simulink model "combinedTxRx_16bit"  (R2017a)
settings: Solver=FixedStepDiscrete  StartTime=0.0  StopTime=10.0  RelTol=1e-3
InitFcn:
  | numHeaderBits = 16;
  | %numPreambleBits = 250;
  | AGCBarkerSymbols = 160+28;
  | EQTrainingSymbols = 250;
  | CRCGeneratorLag = 34; % CRCLen + 2
  | 
  | %% AGC Preamble
  | B13bipolar = [0 0 0 0 0 2 2 0 0 2 0 2];
  | rep = [B13bipolar, B13bipolar(1:4)];
  | AGCBarker = repmat(rep,1,10);
  | % Second preamble part
  | B11bipolar = [0 0 0 2 2 2 0 2  2 0 2];
  | TimingBarker = [B11bipolar,B11bipolar,B11bipolar,B11bipolar(1:6)];
  | PreambleBarkersInts = [AGCBarker, TimingBarker];
  | % Convert integer into their bit representation
  | PreambleBarkersBits = zeros(1,length(PreambleBarkersInts)*2);
  | PreambleBarkersBits(1:2:end) = (PreambleBarkersInts==2);
  | 
  | % Constants
  | % First preamble part
  | B13bipolar = [0 0 0 0 0 2 2 0 0 2 0 2];
  | rep = [B13bipolar, B13bipolar(1:4)];
  | AGCBarker = repmat(rep,1,10);
  | % Second preamble part
  | B11bipolar = [0 0 0 2 2 2 0 2  2 0 2];
  | TimingBarker = [B11bipolar,B11bipolar,B11bipolar(1:6)];
  | PreambleBarkersInts = [AGCBarker, TimingBarker];
  | % Convert integer into their bit representation
  | PreambleBarkersBits = false(1,length(PreambleBarkersInts)*2);
  | PreambleBarkersBits(1:2:end) = logical(PreambleBarkersInts==2);
  | pLen = uint16(length(PreambleBarkersBits));
  | 
  | 
  | %%%%%%%%%%%%%%%%%%%%%%%%%%
  | %% RX
  | %%%%%%%%%%%%%%%%%%%%%%%%%%
  | 
  | barker = comm.BarkerCode('SamplesPerFrame', 28, 'Length', 11);
  | seq = barker()+1;
  | M = 4;
  | hPSKModTrain   = comm.PSKModulator(M, ...
  |     'PhaseOffset',pi/4, ...
  |     'SymbolMapping','Binary');
  | xPreambleSeq = hPSKModTrain(seq);
  | 
  | 
  | %%%%%%%%%%%%
  | 
  | % AGC Preamble
  | reps = 5;
  | barker = comm.BarkerCode('SamplesPerFrame', 16, 'Length', 13);
  | seq = barker()+1;
  | %preamble = zeros(16*reps,1);
  | preambleFull = repmat(seq,reps,1);
  | rctFilt = comm.RaisedCosineTransmitFilter('FilterSpanInSymbols', 128,...
  | 'RolloffFactor',0.5,...
  | 'OutputSamplesPerSymbol',4);
  | preambleFullFilt = rctFilt(preambleFull);
  | 
  | %%%%%%%%%%%%
  | ... (+26 lines)
undefined symbols (not defined in the file or in its folder): j
libraries: simulink x22, dsphdlfiltering x20, hdlsllib x6, commseqgen3 x4, dspsigops x4, commdigbbndpm3 x3, commcrc2 x2, commcnvcod2 x2, dspstat3 x2, commsource2 x1, commutil2 x1, commfilt2 x1
(part 3 of 3)

== matlab function combinedTxRx_16bit/Combined TX and RX/Tx Under Test/Transmitter HDL/Packet Generation/Tx Controller ==
  data: modeOut output; headerData output; data output; payloadBit input; payloadSize input; count input; start input; dataStart output; dataEnd output; preambleReset output
function [modeOut, headerData, data, dataStart, dataEnd, preambleReset] = fcn(payloadBit,payloadSize,count, start)

% When we get a start flag buffers are reset and the next cycle with start
% in mode 0

% Reset: New payload size is passed at an int16
% 


persistent  headerBits numPayloadBits mode

numHeaderBits = uint32(16);
AGCBarkerSymbols = 160+28;
EQTrainingSymbols = 250; % 2 bits per symbol => 250 symbols
preambleBits = uint32(EQTrainingSymbols+AGCBarkerSymbols-0);
CRCLength = 32;
CRCGeneratorLag = CRCLength+2+0; % additional 1 is from reset of encoder
CodeRate = 2;
lagBits = 40+68;

% Async/Init
if isempty(numPayloadBits)
    % Sizes of frame sections
    numPayloadBits = uint32(0); 
    %headerBits = zeros(1,numHeaderBits)>0;
    headerBits = uint16(0);
    mode = uint8(4);
end

% Synchronous
switch mode
    case uint8(0) % Reset
        % Move to next mode on next input/clock
        mode = uint8(1);
        % Convert payloadSize to bits
        numPayloadBits = uint32(bitshift(payloadSize,3)+CRCLength);
        %headerBits = logical(bitget(CodeRate*(payloadSize+CRCLength),1:numHeaderBits));
        headerBits = uint16(bitshift((bitshift(payloadSize,3)+CRCLength+lagBits),1));        
        % Set outputs
        modeOut = uint8(4);
        headerData = false;
        data = false; % Not used downstream
        dataStart = false;
        dataEnd = false;
        preambleReset = true;
    case uint8(1) % Preamble
        % Set Next Mode
        if count>=(preambleBits)
            preambleReset = false;
            mode = uint8(2);
        elseif count==uint32(1)
            preambleReset = false;
            mode = uint8(1);
        else
            preambleReset = false;
            mode = uint8(1);
        end
        % Set outputs
        modeOut = uint8(1);
        headerData = false;
        % Start outputing data early to compensate for CRC lag
        if count>=(preambleBits+numHeaderBits-CRCGeneratorLag)
           data = payloadBit;
           % Set flag on first payload bit
           dataStart = count == (preambleBits+numHeaderBits-CRCGeneratorLag);
        else
           data = false;         
           dataStart = false;
        end
        dataEnd = false;
    case uint8(2) % Header bits
        % Set Next Mode
        if count>=(preambleBits+numHeaderBits)
            mode = uint8(3);
        else
            mode = uint8(2);
        end
        % Set outputs
        modeOut = uint8(2);
        %headerData = headerBits(count-preambleBits);
        headerData = bitget(headerBits,count-preambleBits)>0;
        data = payloadBit;
        dataStart = false;
        dataEnd = false;
        preambleReset = false;
    case uint8(3) % Payload bits and CRC
        % Set Next Mode
        if count>=(preambleBits+numHeaderBits+numPayloadBits)%+CRCGeneratorLag)
            % Will coencide with last CRC Bit
            mode = uint8(4);
        else
            mode = uint8(3);
        end
        % Set outputs
        modeOut = uint8(3);        
        headerData = false;
        data = payloadBit;
        % Set flag on last payload bit
        dataStart = false;
        dataEnd =   ( count==(preambleBits+numHeaderBits+numPayloadBits-CRCLength-CRCGeneratorLag-1) );
        preambleReset = false;
    otherwise %case uint8(4) % Waiting for data
        % Chilling for new start
        if start
           mode = uint8(0); 
        else
           mode = uint8(4);
        end
        % Set outputs
        modeOut = uint8(4);
        headerData = false;
        data = false; % Not used downstream
        dataStart = false;
        dataEnd = false;
        preambleReset = false;
end

== matlab function combinedTxRx_16bit/Combined TX and RX/Tx Under Test/Transmitter HDL/DMA Interface/DMA Control ==
  data: byteIn input; bitOut output; validIn input; validOut output; startOut output; payloadLength output; readyForInput output; EOF input
function [bitOut,validOut,startOut,payloadLength,readyForInput] = DMA_Control(byteIn,validIn,EOF)

% This block converts the byte input pipeline into bits and extract the
% length the packet into its own signal

persistent wordBuffer bitCounter payloadLenBuff mode inputByteCounter

bitsInInput = uint8(16);

if isempty(wordBuffer)
    wordBuffer = uint16(0); % Must match number of bits defined by bitsInInput
    bitCounter = uint8(0);
    payloadLenBuff = uint16(0);
    mode = uint8(0);
    inputByteCounter = uint16(0);
end

%% Payload length setup
% Capture first payload length byte(s)
if validIn && mode == uint8(0)
    bitOut = false;
    validOut = false;
    startOut = true;
    payloadLength = uint16(0);
    readyForInput = true;
    mode = uint8(2);
    inputByteCounter = uint16(0);% Reset
    
    %payloadLenBuff = bitshift(uint16(byteIn),8); % Place upper bits first
    payloadLenBuff = uint16(byteIn); 
    

%% Payload output
% Byte edge of data
elseif validIn && (mode==uint8(2))
    bitOut = bitget(byteIn,1)>0;
    wordBuffer = byteIn; % Save byte
    bitCounter = uint8(2);% Reset
    validOut = true;
    startOut = false;
    readyForInput = false;
    payloadLength = uint16(payloadLenBuff);
    % Bytes processed
    inputByteCounter = inputByteCounter + uint16(bitsInInput/8);    
    
% Remaining N-1 bits of input byte(s)
elseif (bitCounter > uint8(0))  && (mode==uint8(2))
    bitOut = bitget(wordBuffer,bitCounter)>0;
    startOut = false;
    payloadLength = uint16(payloadLenBuff);
    validOut = true;
    if bitCounter >= uint8(bitsInInput)
        bitCounter = uint8(0);
        % If we've processed all the bytes we need to wait for downstream
        % to be done
        if inputByteCounter<payloadLenBuff
            readyForInput = true; % Tell them we need next byte
        else
            readyForInput = false; % Hold DMA off for now, next call will go to EOF
            mode = uint8(3);
        end
    else
        bitCounter = bitCounter+uint8(1);
        readyForInput = false;
    end
% Waiting for EOF from packet generation
elseif (mode==uint8(3))
    bitOut = false;
    validOut = true; % Keep downstream processing going
    startOut = false;
    payloadLength = uint16(payloadLenBuff);
    if EOF % Done with frame now ask for more data
        readyForInput = true;
        mode = uint8(0);% Reset
    else
        readyForInput = false;
    end
    
else % not-valid and need another byte
    bitOut = false;
    if mode == uint8(0)
        validOut = true; % Let LFSR Run
    else
        validOut = false;
    end
    startOut = false;
    payloadLength = uint16(0);
    readyForInput = true;
end

== matlab function combinedTxRx_16bit/Combined TX and RX/Tx Under Test/Transmitter HDL/Packet Generation/Payload/HDL Scrambler 2 bits/Buffer Manage ==
  data: bit1 input; bit2 input; outBuffer output; reset input
function outBuffer = fcn(bit1, bit2, reset)
%#codegen

init_buffer = logical([0 1 0 0 0 1 0]);

persistent buffer

if isempty(buffer)
    buffer = init_buffer;
end

if reset
    outBuffer = init_buffer;
    buffer = init_buffer;
    %outBuffer = [init_buffer(3:end),bit1,bit2];
    %buffer = [buffer(3:end),bit1,bit2];    
else
    outBuffer = [bit2,bit1,buffer(1:end-2)];
    buffer = [bit2,bit1,buffer(1:end-2)];
end

== matlab function combinedTxRx_16bit/Combined TX and RX/Tx Under Test/DMA Model Driver ==
  data: driver input; payload output; valid output boolean; enable input
function [payload,valid] = fcn(driver, enable)
%#codegen

persistent indx mode

pSize = uint16(200); % Size in bytes (Must be multiple of 32 bits) cannot exceed uint16 max
mask = uint16(sum(2.^(0:15)));

if isempty(indx)
    indx = pSize;
    mode = int8(0);
end

% % Randomly dont transmit new data
% if enable && mode == 0
%    enable = randn>1; 
% end

if enable && driver
    valid = true;
    switch mode
        case int8(0) % Fresh packet start
%             disp('New Packet Start');
            payload = uint16(pSize);%Upper bits
            mode = int8(1);
            indx = uint16(0);
        otherwise%case 2
            indx = indx + uint16(2);
            %payload = uint32(sum(2.^[0 2 4 6 8 10 12 14 ]));
            payload = uint16(21845);%sum(2.^[0:2:14])); % Alternating ones and zeros
            if indx == pSize % reached end of frame
                mode = int8(0);
            end
    end
else
    valid = false;
    payload = uint16(0);
end

== matlab function combinedTxRx_16bit/Combined TX and RX/Receiver HDL/CRC Check and DMA Pack/CRC Check ES/Check CRC Result (DEBUG) ==
  data: bits input; start input; done input; valid input; err input
function fcn(bits, start, done, valid, err)

persistent buffer

if isempty(buffer)
    buffer = fi(false(1032,1),0,1,0);
end

buffer = [buffer(2:end);bits];

if done && valid
    if err
        fprintf('CRC Error (HDL CRC)\n');
    else
        fprintf('CRC Passed (HDL CRC)\n');
    end
end
if err % Flag if any error every occurs, if it occurs alone it means given crc is not long enough
    fprintf('CRC Error Type 2 (HDL CRC)\n');
end

== matlab function combinedTxRx_16bit/Combined TX and RX/Receiver HDL/CRC Check and DMA Pack/CRC Check ES/Debug CRC input ==
  data: u input; enable input; endFlag input; startFlag input
function fcn(u, enable,endFlag,startFlag)

persistent buffer crc count

if isempty(buffer)
   buffer = false(1700,1); 
    crc = comm.CRCDetector('Polynomial','z^32 + z^26 + z^23 + z^22 + z^16 + z^12 + z^11 + z^10 + z^8 + z^7 + z^5 + z^4 + z^2 + z + 1');
    count = 1;
end

if enable
    %buffer = [buffer(2:end);u];
    if startFlag
        count = 1;
    elseif count>1700-1
        count = 1;
    else
        count = count + 1;
    end
    buffer(count) = u;
    
    if endFlag
        disp(count)
        k = buffer(1:1632);
        [~,e] = crc(k);
        if e
            disp('Error');
        else
            disp('Pass');
        end
    end
    
end

== matlab function combinedTxRx_16bit/Combined TX and RX/Receiver HDL/CRC Check and DMA Pack/DMA Interface/Bit Packer ==
  data: bitIn input; byteOut output; startIn input; endIn input; err input; validIn input; validOut output; startOut output
function [byteOut,validOut,startOut] = BitPacker(bitIn, startIn, endIn, err, validIn)

% This block will pack bits into bytes with start boundaries


% Constants
bits2Pack = uint8(16); % byteReg must contain this many bits
% NOTE: Frames but be a multiple of bits2Pack or bits will be trimmed from
% end

persistent byteReg byteIndx setStartFlag

if isempty(byteIndx)
    byteReg  = uint16(0);
    byteIndx = uint8(1);
    setStartFlag = false;
end

if validIn
    if startIn % Reset
        bitset(byteReg,1,bitIn);
        byteIndx = uint8(2);
        validOut = false;
        setStartFlag = true;
        startOut = false;
    else
        byteReg = bitset(byteReg,byteIndx,bitIn);
        if byteIndx >= bits2Pack
            byteIndx = uint8(1);
            validOut = true;
            startOut = setStartFlag;
            setStartFlag = false;
        else
            byteIndx = byteIndx + uint8(1);
            validOut = false;
            startOut = false;
        end
    end
elseif endIn % Append error bit to last byte
    byteReg = uint16(err);
    validOut = true;
    startOut = false;
else
    validOut = false;
    startOut = false;
end

byteOut = byteReg;

== matlab function combinedTxRx_16bit/Combined TX and RX/Receiver HDL/CRC Check and DMA Pack/overdrive ==
  data: validIn input; enableCRC output; endIn input
function enableCRC = fcn(validIn,endIn)

% This block drives the enabled subsystem and additional step so the
% outputs do not stay high but reset.  All signals are reset since the
% driving valid signal is false

persistent gotEndOut

if isempty(gotEndOut)
    gotEndOut = false;
end
    
if validIn
    enableCRC = true;
    gotEndOut = false;
else
    if endIn
        gotEndOut = true;
        enableCRC = true;
    elseif gotEndOut
        enableCRC = true;
    else
        enableCRC = false;
    end
end

== matlab function combinedTxRx_16bit/Combined TX and RX/Receiver HDL/Descramble and Decode/Find packet tail and check CRC (DEBUG ONLY) ==
  data: u input; enable output; crcCase output
function [enable, crcCase]=findTail(u)

persistent tailBits buffer counter head

if isempty(tailBits)
   tailBits = repmat(uint8([1 0 1 1 0 0 1 1 1 1].'),4,1);
   buffer = uint8(zeros(size(tailBits)));
    counter = 0;
    head = uint8(ones(16,1));
end

%buffer = [u; buffer(1:end-1)];
buffer = [buffer(2:end); u];
counter = counter + 2; % Coded bit counter

% Check for tail sequence
found = 0;
if isequal(buffer,tailBits)
   fprintf('Found tail after %d coded bits\n',int64(counter));
   counter = 0;
   found = 1;
end

%% CHECK CRC
persistent crc buffer2
CRCLen = 32;
nPayLoad = 8*200;
nTB = length(tailBits);

if isempty(crc)
    crc = comm.CRCDetector('Polynomial','z^32 + z^26 + z^23 + z^22 + z^16 + z^12 + z^11 + z^10 + z^8 + z^7 + z^5 + z^4 + z^2 + z + 1');
    buffer2 = false(CRCLen+nPayLoad+nTB,1);%false(10532+40,1);
end

crcCase = 0;
enable = false;

buffer2 = [buffer2(2:end); u>0];
%if isequal(head, buffer2(end-15:end))
%   fprintf('Head FOUND %d\n',int64(counter));
%end
if found>0
    NoTailBits = buffer2(1:end-nTB);
    PayloadWithCRC= NoTailBits(end-nPayLoad-CRCLen+1:end);
    enable = true;
    [~,e] = crc(PayloadWithCRC);
    if ~e
        crcCase = 1;
        fprintf('Packet CRC Passed\n');
    else
        crcCase = 0;
        fprintf('Packet CRC Failed\n');
    end
    
end

== matlab function combinedTxRx_16bit/Combined TX and RX/Receiver HDL/Frame Recover/Enable Equalizer and Packet Decode (Latch) ==
  data: start input; enable output; validIn input
function enable = Counter(start,validIn)

persistent count maxCount lastEOF

if isempty(count)
    count = uint32(0);
    maxCount = uint32(2^16); % Largest possible packet length
    lastEOF = false;
end

eof = false;

if validIn
    % Got a barker preamble start allowing data into equalizer
    if start
        count = maxCount;
    end
    
    % Check on change from true to false
    if lastEOF && ~eof
        %     fprintf('Frame end reached\n');
        count = uint32(0);
    end
    lastEOF = eof;
    
    % Past end of max frame size
    if count>0
        count = count - uint32(1);
    end
    
    % Enable downstream
    enable = count>uint32(0);
else
    enable = false;
end

== matlab function combinedTxRx_16bit/Combined TX and RX/Receiver HDL/Frame Recover/Equalization and Demodulation/2 Bit Descrambler/MATLAB Function ==
  data: bits input; bufferA output; reset input; bufferB output
function [bufferA, bufferB] = BufferSelect(bits,reset)

persistent buffer

% Constants
initBuffer = logical([0 1 0 0 0 1 0]);

% Async
if isempty(buffer)
    buffer = initBuffer;
end

% Reset/Sync
if reset
    bufferA = initBuffer;
    bufferB = [bits(1),initBuffer(1:end-1)];
    buffer = [bits(2),bits(1),initBuffer(1:end-2)];
else
    bufferA = buffer;
    bufferB = [bits(1),buffer(1:end-1)];
    buffer = [bits(2),bits(1),buffer(1:end-2)];    
end

== matlab function combinedTxRx_16bit/Combined TX and RX/Receiver HDL/Frame Recover/Equalization and Demodulation/DFE/Equalizer ==
  data: trigger input; eqOut output; data input; trainingSymbol input
function eqOut  = dfe(trigger,data,trainingSymbol)

persistent inputBuffer decisionBuffer forwardTaps backwardTaps processedSamples


%% Constants
WL = uint8(16); FL = uint8(14);
F = fimath('SumMode','SpecifyPrecision','SumWordLength',WL,...
    'SumFractionLength',FL);
% Initial delay guess
channelDelay = uint8(0);
% Equalizer settings
mu = fi(0.05,0,10,12);
nFTaps = uint8(11);
nBTaps = uint8(3);
numTrainingSymbols = uint16(250);
resetTaps = fi([complex(zeros(nFTaps-1,1));1],1,WL,FL,F);

%% Async
if isempty(inputBuffer)
    % Set Precisions
    inputBuffer = fi(complex(zeros(nFTaps,1)),1,WL,FL,F);
    decisionBuffer = fi(complex(zeros(nBTaps,1)),1,WL,FL,F);
    forwardTaps = fi(complex(zeros(nFTaps,1)),1,WL,FL,F);
    backwardTaps = fi(complex(zeros(nBTaps,1)),1,WL,FL,F);
    processedSamples = numTrainingSymbols + uint16(1); % Force to DD mode to start
end

%% Reset
if trigger
    processedSamples = uint16(0);
    % Reset taps
    %forwardTaps = fi(complex(zeros(nFTaps,1)),1,WL,FL,F);
    %forwardTaps(nFTaps-channelDelay) = fi(1,1,WL,FL); % Favor specific delay (causes equalizer to converge faster)
    forwardTaps = resetTaps;
    backwardTaps = fi(complex(zeros(nBTaps,1)),1,WL,FL,F);
    % Default output
    eqOut = fi(0,1,WL,FL,F);
else
    %% Equalizer
    % Add data to buffer
    inputBuffer = [inputBuffer(2:end);data];
    
    % Apply equalizer
    eqOut = forwardTaps'*inputBuffer - backwardTaps'*decisionBuffer;
    
    % Determine error
    if (processedSamples<numTrainingSymbols) && (processedSamples>=channelDelay)
        processedSamples = processedSamples + 1;
        d = trainingSymbol;
    else % Decision directed
        % Find closest symbol
        r = real(eqOut)>0; i = imag(eqOut)>0;
        if r
            if i
                d = fi(0.7071 + 0.7071i,1,WL,FL);
            else
                d = fi(0.7071 - 0.7071i,1,WL,FL);
            end
        else
            if i
                d = fi(-0.7071 + 0.7071i,1,WL,FL);
            else
                d = fi(-0.7071 - 0.7071i,1,WL,FL);
            end
        end
    end
    ec = conj(d - eqOut);
    
    % Update taps
    forwardTaps = forwardTaps + mu*ec*inputBuffer;
    backwardTaps = backwardTaps - mu*ec*decisionBuffer;
    
    % Update decision buffer
    db = fi(d,1,WL,FL,F);
    decisionBuffer = [db; decisionBuffer(1:end-1)];
    
end



end

== matlab function combinedTxRx_16bit/Combined TX and RX/Receiver HDL/Frame Recover/Equalization and Demodulation/Header Controller ==
  data: headerStart input; enableDownstream output; packetLenBitsOut output; data input; resetViterbi output; crcStart output
function [enableDownstream,packetLenBitsOut,resetViterbi,crcStart] = EvalHeader(headerStart, data)

persistent counter sum1 sum2 packetLenBits lastMode savedPacketLenBits

% The header contains 16 bits, but each bit is duplicated to make checking
% easier

% Note this block works on symbols (2bits) but 1 symbol -> 1 decoded bit

% PacketLength = (Data+CRC+40(TB)+68)/CodeRate

% NOTE TAIL BITS HERE ARE REALLY USED TO DEAL WITH VITERBI LAG SO:
% TailBitsWithLagPadding > TracebackLength

%% Constants
numHeaderBits = uint8(16); % Header is this many bits
powersOfTwo = uint32([1 2 4 8 16 32 64 128 256 512 1024 2048 4096 8192 16384 32768]);
%TracebackLength = uint32(34)+uint32(20);
%CRCLen = uint32(32);
CodeRateINV = uint32(2);%1/CodeRate;
TailBitsWithLagPadding = uint32(uint32(40)+34*2+1);
% Flag when CRC porition of packet starts relative to header
%crcSignalStartLocation = uint32((TailBitsWithLagPadding+CRCLen)*CodeRateINV); % Must be even
crcSignalStartLocation = uint32((TailBitsWithLagPadding)*CodeRateINV); % Must be even

% Async
if isempty(counter)
    packetLenBits = uint32(0);
    sum1 = uint32(0);
    sum2 = uint32(0);
    counter = uint8(numHeaderBits);
    lastMode = uint8(3);
    savedPacketLenBits = uint16(0);
end

%% Sync
% Got a header now enable certain mode
if headerStart
    mode = uint8(0);
else
    mode = lastMode;
end

switch mode
    %% Reset on preamble flag and setup for header processing
    case uint8(0)
        crcStart = false;
        resetViterbi = false;
        enableDownstream = false;
        sum1 = uint32(0);
        sum2 = uint32(0);
        counter = uint8(1);
        lastMode = uint8(1); % Go to next state
        packetLenBitsOut = uint16(0);
        
    %% Process header
    case 1 
        crcStart = false;
        enableDownstream = false; %%%%%%%%%%% CHECK!
        
        % Convert header bits (bit by bit)
        if data(1)
            sum1 = sum1 + powersOfTwo(counter);
        end
        if data(2)
            sum2 = sum2 + powersOfTwo(counter);
        end
        counter = counter + uint8(1);
        
        if counter>numHeaderBits
            % Check header
            if sum1~=sum2 % Fail
                packetLenBits = uint32(0);
                lastMode = uint8(3);
                resetViterbi = false;
                packetLenBitsOut = uint16(0);
                savedPacketLenBits = uint16(0);
%                 fprintf('Header Check failed (possible false detection)\n');
%                 fprintf('sum1: %d\n',int32(sum1));
%                 fprintf('sum2: %d\n',int32(sum2));
            else % Pass
                % Saved header info and trigger downstream
                packetLenBits = uint32(sum1);
                lastMode = uint8(2);
                resetViterbi = true;
                packetLenBitsOut = uint16(sum1-crcSignalStartLocation);
                savedPacketLenBits = uint16(sum1-crcSignalStartLocation);
%                 fprintf('Header Found | Packet is %d bits long\n',int32(sum1));            
            end
        else
            packetLenBitsOut = uint16(0);
            resetViterbi = false;
        end
        
    %% Decrement sample counter
    case 2 
        resetViterbi = false;
        crcStart = (packetLenBits==crcSignalStartLocation);
        if packetLenBits>uint32(0)
            enableDownstream = true;
            packetLenBits = packetLenBits - uint32(2); % We get 2 bits each call
            packetLenBitsOut = savedPacketLenBits;
        else
            enableDownstream = false;
            lastMode = uint8(3);
            packetLenBitsOut = uint16(0); %Reset
            savedPacketLenBits = uint16(0);%Reset
        end
            
    %% Not processing anything
    otherwise % mode>2
        crcStart = false;
        resetViterbi = false;
        enableDownstream = false;
        packetLenBitsOut = uint16(0);
end

%%

% % Set default flags, which may change
% resetViterbi = false;
% crcStart = false;
% 
% % Reset when preamble found (barker sequence)
% if headerStart
%     sum1 = uint32(0);
%     sum2 = uint32(0);
%     counter = uint32(1);
% end
% 
% % Send data downstream to
% enableDownstream = packetLenBits>uint32(0);
% 
% % Flag when we are in CRC section of packet
% % Enable signal will relate to first bit of CRC portion of packet
% if packetLenBits==crcSignalStartLocation
%     crcStart = true;
% end
% 
% % Decrement packet length counter
% if enableDownstream
%     packetLenBits = packetLenBits - uint32(2); % Get 2 bits each call
% end
% 
% % Process header
% if counter<=headerBits
%     % Convert header bits (bit by bit)
%     if data(1)
%         sum1 = sum1 + powersOfTwo(counter);
%     end
%     if data(2)
%         sum2 = sum2 + powersOfTwo(counter);
%     end
%     counter = counter + uint32(1);
%     
%     if counter>headerBits
%         % Check header
%         if sum1~=sum2
%             packetLenBits = uint32(0);
%             enableDownstream = false;
%             fprintf('Header Check failed (possible false detection)\n');
%         else
%             % Saved header info and trigger downstream
%             packetLenBits = uint32(sum1);
%             fprintf('Header Found | Packet is %d bits long\n',int32(sum1));
%             resetViterbi = true;
%             enableDownstream = true;
%         end
%     end
%     
% end

== matlab function combinedTxRx_16bit/Combined TX and RX/Receiver HDL/Frame Recover/Equalization and Demodulation/MATLAB Function ==
  data: d1 input; d2 input
function fcn(d1, d2)


if isequal(d1,d2) && ~isequal(d1,zeros(16,1))
    disp('Equal');
end

== matlab function combinedTxRx_16bit/Combined TX and RX/Receiver HDL/Frame Recover/Equalization and Demodulation/MATLAB Function1 ==
  data: start input; qpsk input; bits input
function fcn(start,qpsk, bits)

persistent buffer buffer2 HeaderDataPad count

if isempty(buffer)
    buffer = complex(zeros(16,1));
    buffer2 = false(32,1);
    
    HeaderLen = 16; % Bits
    %PayloadCodedLen = (length(frame)+0)/rate;
    PayloadCodedLen = 3480;
    HeaderData = bitget(PayloadCodedLen,1:HeaderLen).';
    
    % Repeatatively encode bits
    HeaderDataPad = reshape([HeaderData HeaderData].',1,HeaderLen*2).';
    count = 0;
end

if start
    disp('start');
    count = 0;
end
count = count + 1;
buffer = [buffer(2:end);double(qpsk)];
buffer2 = [buffer2(3:end);bits(:)];
if isequal(HeaderDataPad,buffer2)
    disp('Found');
end

== matlab function combinedTxRx_16bit/Combined TX and RX/Receiver HDL/Frame Recover/Frequency Recovery/Loop Filter/Flip Sign ==
  data: u input; y output
function y = fcn(u)

WL = 25;
FP = 20;

% Flip sign x = (~y) + 1
u8 = bitcmp(int8(u));
y = fi(u8+int8(1),1,WL,FP);

== matlab function combinedTxRx_16bit/Combined TX and RX/Receiver HDL/Frame Recover/Frequency Recovery/PED ==
  data: In input; e output
function e  = PED(In)

OP2 = real(In);
OP1 = imag(In);

Real = OP2;
Imag = OP1;

if (bitget(Real,16)==true) % real component is negative
    OP1 = fi(-Imag,1,16,13);
end
if (bitget(Imag,16)==true) % imaginary component is negative
    OP2 = fi(-Real,1,16,13);
end

e= fi(OP1-OP2,1,16,10);

%e = sign(real(In)).*imag(In) - sign(imag(In)).*real(In);
